simulink model "PWR"  (R2019b)
settings: Solver=VariableStepAuto  StartTime=0.0  StopTime=3  RelTol=1e-3  EnableMultiTasking=on
values from neighbouring files (symbols this model uses):
  A = 0.93    [PWR_params.m]
  C = 40e-6    (= 4e-05)    [PWR_params.m]
  E = 670    [PWR_params.m]
  K_vco = 250    [PWR_params.m]
  L = (400e-6)/2    (= 0.0002)    [PWR_params.m]
  omega_ref = 50    [PWR_params.m]
  omega_vco_free = omega_ref - 146.37/2/pi    (= 26.7044909796)    [PWR_params.m]
  R = 1.22    [PWR_params.m]
  tau_1 = 0.0448    [PWR_params.m]
  tau_2 = 0.0185    [PWR_params.m]
  x_0 = -0.032    [PWR_params.m]
libraries: powerlib x30, powerlib_meascontrol x3, eeTransforms x1
settings Model: Creator=Dmitry Sorokin  LastModifiedBy=mir
settings DataIOCC: LimitDataPoints=on  ReturnWorkspaceOutputs=off
settings OptimizationCC: LifeSpan=inf
settings DebuggingCC: AllowSymbolicDim=off  SFUnexpectedBacktrackingDiag=warning  SFNoUnconditionalDefaultTransitionDiag=warning  SFExecutionAtInitializationDiag=none  ArithmeticOperatorsInVariantConditions=warning
settings ModelReferenceCC: PropagateSignalLabelsOutOfModel=off
settings SFSimCC: SimUseLocalCustomCode=off  CustomCodeUndefinedFunction=UseInterfaceOnly
settings RTWCC: RTWUseLocalCustomCode=off
settings CodeAppCC: StateflowObjectComments=on
settings GRTTargetCC: TargetLangStandard=C89/C90 (ANSI)
settings ConfigComp: CovMetricSettings=dw  CovHtmlReporting=on  CovSaveCumulativeToWorkspaceVar=on  CovSaveSingleToWorkspaceVar=on  CovExternalEMLEnable=off
settings SimscapeCC: SimscapeNormalizeSystem=off

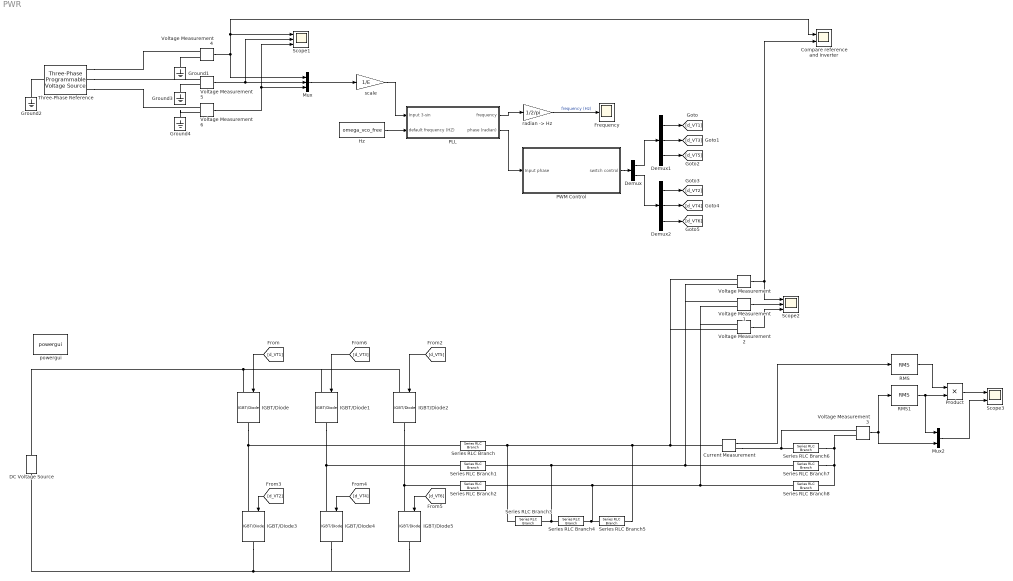
== system PWR ==
  Compare reference and inverter : Scope  NumInputPorts=2
  Current Measurement : powerlib/Measurements/Current Measurement  PhasorSimulation=off  OutputType=Complex  PSBequivalent=0
      settings: SourceProductName=Simscape Electrical
  DC Voltage Source : powerlib/Electrical Sources/DC Voltage Source  Amplitude=E  Measurements=None
      settings: SourceProductName=Simscape Electrical
  Demux : Demux  Outputs=2
  Demux1 : Demux  Outputs=3
  Demux2 : Demux  Outputs=3
  Frequency : Scope
  Ground{1..4} (4 alike) : powerlib/Elements/Ground  LConnTagsString=a
      settings: SourceProductName=Simscape Electrical
  Hz : Constant  Value=omega_vco_free
  IGBT/Diode{,1..5} (6 alike) : powerlib/Power Electronics/IGBT//Diode  Ron=1e-3  Rs=1e5  Cs=inf  Measurements=off
      settings: SourceProductName=Simscape Electrical
  Mux : Mux  Inputs=3
  Mux2 : Mux  Inputs=2
  PLL : Subsystem
  PWM Control : Subsystem
  Product : Product
  RMS : powerlib_meascontrol/Measurements/RMS  TrueRMS=on  Freq=50  RMSInit=120  Ts=0
      settings: SourceProductName=Simscape Electrical
  RMS1 : powerlib_meascontrol/Measurements/RMS  TrueRMS=on  Freq=50  RMSInit=120  Ts=0
      settings: SourceProductName=Simscape Electrical
  Scope1 : Scope  NumInputPorts=3
  Scope2 : Scope  NumInputPorts=3
  Scope3 : Scope  NumInputPorts=2
  Series RLC Branch : powerlib/Elements/Series RLC Branch  LConnTagsString=__new0  RConnTagsString=__new0  BranchType=L  Resistance=1  Inductance=L  SetiL0=off  InitialCurrent=0  Capacitance=1e-6  Setx0=off  InitialVoltage=0  Measurements=None
      settings: SourceProductName=Simscape Electrical
  Series RLC Branch1 : powerlib/Elements/Series RLC Branch  LConnTagsString=__new0  RConnTagsString=__new0  BranchType=L  Resistance=1  Inductance=L  SetiL0=off  InitialCurrent=0  Capacitance=1e-6  Setx0=off  InitialVoltage=0  Measurements=None
      settings: SourceProductName=Simscape Electrical
  Series RLC Branch2 : powerlib/Elements/Series RLC Branch  LConnTagsString=__new0  RConnTagsString=__new0  BranchType=L  Resistance=1  Inductance=L  SetiL0=off  InitialCurrent=0  Capacitance=1e-6  Setx0=off  InitialVoltage=0  Measurements=None
      settings: SourceProductName=Simscape Electrical
  Series RLC Branch3 : powerlib/Elements/Series RLC Branch  LConnTagsString=__new0  RConnTagsString=__new0  BranchType=C  Resistance=1  Inductance=1e-3  SetiL0=off  InitialCurrent=0  Capacitance=C  Setx0=off  InitialVoltage=0  Measurements=None
      settings: SourceProductName=Simscape Electrical
  Series RLC Branch4 : powerlib/Elements/Series RLC Branch  LConnTagsString=__new0  RConnTagsString=__new0  BranchType=C  Resistance=1  Inductance=1e-3  SetiL0=off  InitialCurrent=0  Capacitance=C  Setx0=off  InitialVoltage=0  Measurements=None
      settings: SourceProductName=Simscape Electrical
  Series RLC Branch5 : powerlib/Elements/Series RLC Branch  LConnTagsString=__new0  RConnTagsString=__new0  BranchType=C  Resistance=1  Inductance=1e-3  SetiL0=off  InitialCurrent=0  Capacitance=C  Setx0=off  InitialVoltage=0  Measurements=None
      settings: SourceProductName=Simscape Electrical
  Series RLC Branch6 : powerlib/Elements/Series RLC Branch  LConnTagsString=__new0  RConnTagsString=__new0  BranchType=R  Resistance=R  Inductance=1e-3  SetiL0=off  InitialCurrent=0  Capacitance=1e-6  Setx0=off  InitialVoltage=0  Measurements=None
      settings: SourceProductName=Simscape Electrical
  Series RLC Branch7 : powerlib/Elements/Series RLC Branch  LConnTagsString=__new0  RConnTagsString=__new0  BranchType=R  Resistance=R  Inductance=1e-3  SetiL0=off  InitialCurrent=0  Capacitance=1e-6  Setx0=off  InitialVoltage=0  Measurements=None
      settings: SourceProductName=Simscape Electrical
  Series RLC Branch8 : powerlib/Elements/Series RLC Branch  LConnTagsString=__new0  RConnTagsString=__new0  BranchType=R  Resistance=R  Inductance=1e-3  SetiL0=off  InitialCurrent=0  Capacitance=1e-6  Setx0=off  InitialVoltage=0  Measurements=None
      settings: SourceProductName=Simscape Electrical
  Three-Phase Reference : powerlib/Electrical Sources/Three-Phase Programmable Voltage Source  PositiveSequence="[E  0 omega_ref]"  VariationEntity=None  VariationType=Table of time-amplitude pairs  VariationTypeAlt=Step  VariationStep=0.5  VariationRate=10  VariationMagnitude=0.3  VariationFrequency=2  VariationTiming=[1 2]  VariationPhaseA=off  Amplitudes=[1 0.8 1.2 1.0]  TimeValues=[0 0.1 0.15 0.2]  HarmonicGeneration=off  HarmonicA=[3 0.2 -25 0]  HarmonicB=[2 0.15 35 2]  Timing="[0.05  3]"  BusType=swing  Pref=0  Qref=0  Qmin=-inf  Qmax=inf
      settings: SourceProductName=Simscape Electrical
  Voltage Measurement{,1..6} (7 alike) : powerlib/Measurements/Voltage Measurement  PhasorSimulation=off  OutputType=Complex  PSBequivalent=0
      settings: SourceProductName=Simscape Electrical
  powergui : powerlib/powergui  Priority=1  SimulationMode=Discrete  SampleTime=1e-3  frequency=60  Iterations=50  frequencyindice=50  Pbase=100e6  ErrMax=1e-4  UnitsV=kV  UnitsW=MW  buscounter=0  FunctionMessages=off  echomessages=off  EnableUseOfTLC=off  CurrentSourceSwitches=off  DisableSnubberDevices=off  DisableRonSwitches=off  DisableVfSwitches=off  DisplayEquations=off  AutomaticDiscreteSolvers=off  SolverType=Tustin/Backward Euler (TBE)  Interpol=off  ExternalGateDelay=off  methode=off  Ts=10  x0status=blocks  SPID=off  SwTol=0  HookPort=off  NonlinearTolerance=1e-4  nMaxIteration=100  ContinueOnMaxIteration=off  RestoreLinks=warning  ResistiveCurrentMeasurement=off  Frange=[0:2:500]  Ylog=off  Xlog=on  ShowGrid=off  save=off  variable=ZData  structure=0  ZoomFFT=off  StartTime=0.0  cycles=1  DisplayStyle=1  fundamental=60  FreqAxis=off  MaxFrequency=1000  frequencyindicesteady=1  RmsSteady=1  display=off
      settings: SourceProductName=Simscape Electrical
  "radian -> Hz" : Gain  Gain=1/2/pi
  scale : Gain  Gain=1/E
  wires:
  [d_VT1] -> IGBT/Diode/1
  [d_VT3] -> IGBT/Diode1/1
  [d_VT5] -> IGBT/Diode2/1
  [d_VT2] -> IGBT/Diode3/1
  [d_VT4] -> IGBT/Diode4/1
  [d_VT6] -> IGBT/Diode5/1
  Voltage Measurement1/1 -> Scope2/2
  Voltage Measurement/1 -> Compare reference and inverter/2, Scope2/1
  Voltage Measurement2/1 -> Scope2/3
  Voltage Measurement3/1 -> RMS1/1, Mux2/2
  Current Measurement/1 -> RMS/1
  RMS/1 -> Product/1
  RMS1/1 -> Mux2/1, Product/2
  Product/1 -> Scope3/1
  Mux2/1 -> Scope3/2
  scale/1 -> PLL/1("Input 3-sin ")
  "radian -> Hz"/1 -> Frequency/1  "frequency (Hz)"
  PLL/1(frequency) -> "radian -> Hz"/1
  Hz/1 -> PLL/2(default frequency (HZ))
  Voltage Measurement6/1 -> Mux/3, Scope1/3
  Voltage Measurement4/1 -> Scope1/1, Compare reference and inverter/1, Mux/1
  Voltage Measurement5/1 -> Mux/2, Scope1/2
  Mux/1 -> scale/1
  PLL/2(phase (radian)) -> PWM Control/1(Input phase)
  PWM Control/1(switch control) -> Demux/1
  Demux1/1 -> [d_VT1]
  Demux1/2 -> [d_VT3]
  Demux/2 -> Demux2/1
  Demux2/3 -> [d_VT6]
  Demux1/3 -> [d_VT5]
  Demux2/1 -> [d_VT2]
  Demux2/2 -> [d_VT4]
  Demux/1 -> Demux1/1
  connections:
  Series RLC Branch/LConn1 -- IGBT/Diode3/LConn1 -- IGBT/Diode/RConn1
  Series RLC Branch1/LConn1 -- IGBT/Diode4/LConn1 -- IGBT/Diode1/RConn1
  Series RLC Branch2/LConn1 -- IGBT/Diode5/LConn1 -- IGBT/Diode2/RConn1
  IGBT/Diode2/LConn1 -- IGBT/Diode1/LConn1 -- IGBT/Diode/LConn1 -- DC Voltage Source/RConn1
  IGBT/Diode5/RConn1 -- IGBT/Diode4/RConn1 -- IGBT/Diode3/RConn1 -- DC Voltage Source/LConn1
  Series RLC Branch3/RConn1 -- Current Measurement/LConn1 -- Voltage Measurement2/LConn2 -- Voltage Measurement/LConn1 -- Series RLC Branch5/LConn1 -- Series RLC Branch/RConn1
  Series RLC Branch4/RConn1 -- Series RLC Branch7/LConn1 -- Voltage Measurement1/LConn1 -- Voltage Measurement/LConn2 -- Series RLC Branch1/RConn1 -- Series RLC Branch3/LConn1
  Series RLC Branch5/RConn1 -- Voltage Measurement2/LConn1 -- Voltage Measurement1/LConn2 -- Series RLC Branch8/LConn1 -- Series RLC Branch2/RConn1 -- Series RLC Branch4/LConn1
  Series RLC Branch6/RConn1 -- Voltage Measurement3/LConn2 -- Series RLC Branch7/RConn1 -- Series RLC Branch8/RConn1
  Series RLC Branch6/LConn1 -- Voltage Measurement3/LConn1 -- Current Measurement/RConn1
  Ground2/LConn1 -- Three-Phase Reference/LConn1
  Three-Phase Reference/RConn1 -- Voltage Measurement4/LConn1
  Three-Phase Reference/RConn2 -- Voltage Measurement5/LConn1
  Three-Phase Reference/RConn3 -- Voltage Measurement6/LConn1
  Ground1/LConn1 -- Voltage Measurement4/LConn2
  Ground3/LConn1 -- Voltage Measurement5/LConn2
  Ground4/LConn1 -- Voltage Measurement6/LConn2

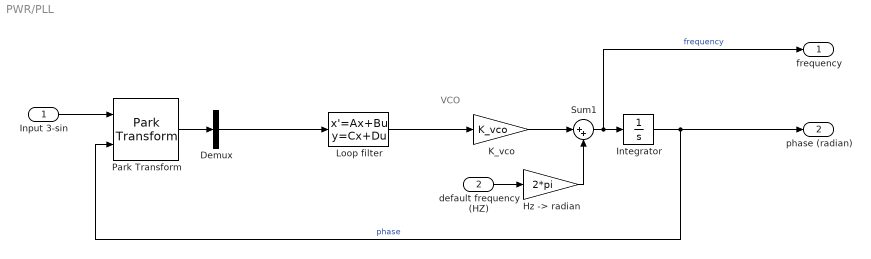
== system PWR/PLL ==
  note: VCO
  "Input 3-sin " : Inport
  default frequency (HZ) : Inport  Port=2
  Demux : Demux  Outputs=3
  "Hz -> radian" : Gain  Gain=2*pi
  Integrator : Integrator
  K_vco : Gain  Gain=K_vco
  Loop filter : StateSpace  A=-1/(tau_1+tau_2)  B=tau_1/(tau_1+tau_2)  C=1/(tau_1+tau_2)  D=tau_2/(tau_1+tau_2)  InitialCondition=x_0
  Park Transform : eeTransforms/Park Transform  AxisAlignment=Q-axis  PowerInvariant=off
      settings: SourceProductName=Simscape Electrical
  Sum1 : Sum  Inputs=|++
  frequency : Outport
  phase (radian) : Outport  Port=2
  wires:
  K_vco/1 -> Sum1/1
  "Hz -> radian"/1 -> Sum1/2
  Integrator/1 -> Park Transform/2, phase (radian)/1  "phase"
  Sum1/1 -> frequency/1, Integrator/1  "frequency"
  Loop filter/1 -> K_vco/1
  Demux/2 -> Loop filter/1
  default frequency (HZ)/1 -> "Hz -> radian"/1
  "Input 3-sin "/1 -> Park Transform/1
  Park Transform/1 -> Demux/1

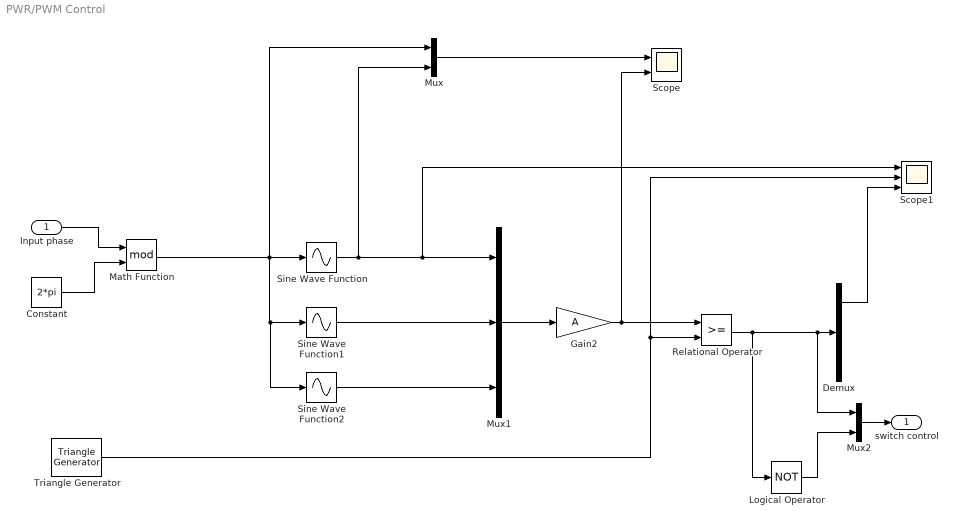
== system PWR/PWM Control ==
  Input phase : Inport
  Constant : Constant  Value=2*pi
  Demux : Demux  Outputs=3
  Gain2 : Gain  Gain=A
  Logical Operator : Logic  Operator=NOT  AllPortsSameDT=off  OutDataTypeStr=boolean
  Math Function : Math  Operator=mod  SignedPower=off  SaturateOnIntegerOverflow=on
  Mux : Mux  Inputs=2
  Mux1 : Mux  Inputs=3
  Mux2 : Mux  Inputs=2
  Relational Operator : RelationalOperator  OutDataTypeStr=boolean  RndMeth=Nearest
  Scope : Scope  NumInputPorts=2
  Scope1 : Scope  NumInputPorts=3
  Sine Wave Function : Sin  TimeSource=Use external signal  SampleTime=0
  Sine Wave Function1 : Sin  TimeSource=Use external signal  Phase=-2*pi/3  SampleTime=0
  Sine Wave Function2 : Sin  TimeSource=Use external signal  Phase=2*pi/3  SampleTime=0
  Triangle Generator : powerlib_meascontrol/Pulse & Signal Generators/Triangle Generator  Freq=f_VT  Phase=90  Ts=0
      settings: SourceProductName=Simscape Electrical
  switch control : Outport
  wires:
  Mux/1 -> Scope/1
  Gain2/1 -> Relational Operator/1, Scope/2
  Mux1/1 -> Gain2/1
  Sine Wave Function2/1 -> Mux1/3
  Sine Wave Function1/1 -> Mux1/2
  Demux/1 -> Scope1/3
  Triangle Generator/1 -> Scope1/2, Relational Operator/2
  Logical Operator/1 -> Mux2/2
  Sine Wave Function/1 -> Mux/2, Scope1/1, Mux1/1
  Relational Operator/1 -> Logical Operator/1, Mux2/1, Demux/1
  Mux2/1 -> switch control/1
  Math Function/1 -> Mux/1, Sine Wave Function2/1, Sine Wave Function1/1, Sine Wave Function/1
  Input phase/1 -> Math Function/1
  Constant/1 -> Math Function/2
